simulink model "lab2"  (R2023b)
settings: Solver=VariableStepAuto  StartTime=0.0  StopTime=100  RelTol=1e-3
undefined symbols (not defined in the file): den, num
libraries: simulink x3
settings Model: Creator=nikita  LastModifiedBy=killer

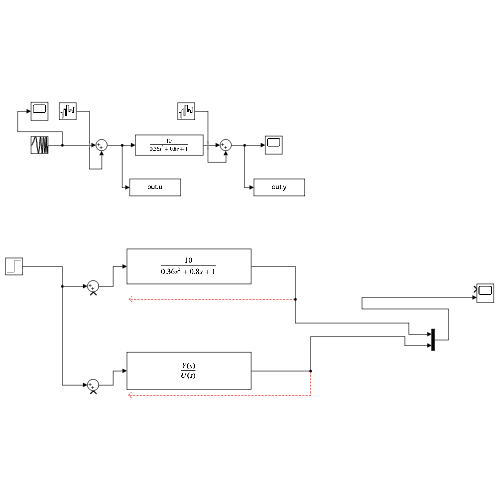
[thumbnail: Simulink's stored preview of the top-level diagram]
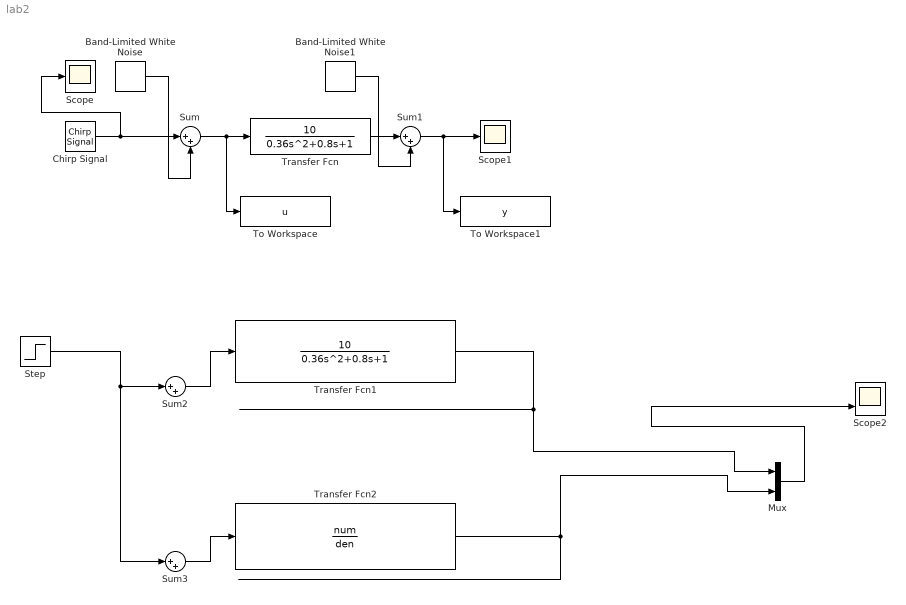
== system lab2 ==
  Band-Limited White Noise : simulink/Sources/Band-Limited White Noise  Cov=[0.1]  Ts=0.1  seed=[23341]
  Band-Limited White Noise1 : simulink/Sources/Band-Limited White Noise  Cov=[0.1]  Ts=0.1  seed=[23341]
  Chirp Signal : simulink/Sources/Chirp Signal  f1=0.1  T=100  f2=1
  Mux : Mux  Inputs=2
  Scope : Scope
  Scope1 : Scope
  Scope2 : Scope  NumInputPorts=2
  Step : Step  SampleTime=0
  Sum{,1..3} (4 alike) : Sum  Inputs=|++
  To Workspace : ToWorkspace  VariableName=u  SaveFormat=Timeseries  SampleTime=-1
  To Workspace1 : ToWorkspace  VariableName=y  SaveFormat=Timeseries  SampleTime=-1
  Transfer Fcn : TransferFcn  Numerator=[10]  Denominator=[0.36 0.8 1]
  Transfer Fcn1 : TransferFcn  Numerator=[10]  Denominator=[0.36 0.8 1]
  Transfer Fcn2 : TransferFcn  Numerator=num  Denominator=den
  wires:
  Chirp Signal/1 -> Scope/1, Sum/1
  Band-Limited White Noise/1 -> Sum/2
  Sum/1 -> To Workspace/1, Transfer Fcn/1
  Transfer Fcn/1 -> Sum1/1
  Band-Limited White Noise1/1 -> Sum1/2
  Sum1/1 -> To Workspace1/1, Scope1/1
  Step/1 -> Sum2/1, Sum3/1
  Transfer Fcn1/1 -> Mux/1
  Sum3/1 -> Transfer Fcn2/1
  Sum2/1 -> Transfer Fcn1/1
  Transfer Fcn2/1 -> Mux/2
  Mux/1 -> Scope2/2
